simulink model "CH12_1"  (R2021b)
settings: Solver=ode45  StartTime=0.0  StopTime=5  RelTol=1e-3
libraries: dsparch4 x2
settings Model: Creator=NA  LastModifiedBy=IT
settings SolverCC: AlgebraicLoopSolver=TrustRegion
settings DataIOCC: LimitDataPoints=on  SaveFormat=Array  SignalLoggingSaveFormat=ModelDataLogs  ReturnWorkspaceOutputs=off
settings OptimizationCC: BlockReduction=off  BooleanDataType=off  LifeSpan=inf
settings DebuggingCC: SaveWithParameterizedLinksMsg=none  UnderspecifiedInitializationDetection=Classic  MergeDetectMultiDrivingBlocksExec=none  SignalResolutionControl=TryResolveAllWithWarning  FcnCallInpInsideContextMsg=warning  SFUnexpectedBacktrackingDiag=warning  SFNoUnconditionalDefaultTransitionDiag=warning  SFExecutionAtInitializationDiag=none  SFMachineParentedDataDiag=warning  ArithmeticOperatorsInVariantConditions=warning
settings HardwareCC: ProdBitPerPointer=32  ProdBitPerSizeT=32  ProdBitPerPtrDiffT=32  ProdLargestAtomicFloat=None  ProdIntDivRoundTo=Undefined  ProdEndianess=Unspecified  ProdWordSize=32  ProdHWDeviceType=32-bit Generic  TargetUnknown=on
settings ModelReferenceCC: PropagateSignalLabelsOutOfModel=off
settings SFSimCC: SimUseLocalCustomCode=off  CustomCodeUndefinedFunction=UseInterfaceOnly
settings RTWCC: RTWUseLocalCustomCode=off
settings CodeAppCC: StateflowObjectComments=on
settings GRTTargetCC: TargetLangStandard=C89/C90 (ANSI)  CombineOutputUpdateFcns=off  GRTInterface=on
settings ConfigComp: CovMetricSettings=dw  CovSaveCumulativeToWorkspaceVar=on  CovSaveSingleToWorkspaceVar=on  CovExternalEMLEnable=off

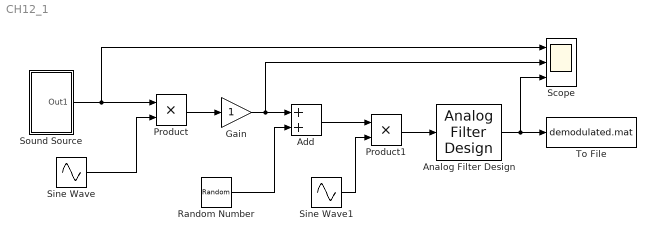
== system CH12_1 ==
  Add : Sum
  Analog Filter Design : dsparch4/Analog Filter Design  method=Butterworth  filttype=Lowpass  N=8  Wlo=2*pi*4e3  Whi=80  Rp=2  Rs=40
  Gain : Gain
  Product : Product
  Product1 : Product
  Random Number : RandomNumber  Variance=1e-6  Seed=41  SampleTime=1/8000  VectorParams1D=off
  Scope : Scope  NumInputPorts=3
  Sine Wave : Sin  Frequency=2*pi*25e3  Phase=pi/2  SampleTime=0
  Sine Wave1 : Sin  Frequency=2*pi*25e3  Phase=pi/2  SampleTime=0
  Sound Source : Subsystem
  To File : ToFile  Filename=demodulated.mat  SampleTime=1/8192
  wires:
  Sound Source/1(Out1) -> Scope/1, Product/1
  Product/1 -> Gain/1
  Gain/1 -> Scope/2, Add/1
  Add/1 -> Product1/1
  Product1/1 -> Analog Filter Design/1
  Analog Filter Design/1 -> Scope/3, To File/1
  Sine Wave/1 -> Product/2
  Random Number/1 -> Add/2
  Sine Wave1/1 -> Product1/2

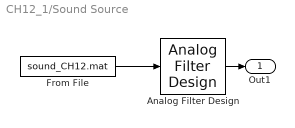
== system CH12_1/Sound Source ==
  Analog Filter Design : dsparch4/Analog Filter Design  method=Butterworth  filttype=Lowpass  N=8  Wlo=2*pi*4e3  Whi=80  Rp=2  Rs=40
  From File : FromFile  FileName=sound_CH12.mat  SampleTime=0
  Out1 : Outport
  wires:
  From File/1 -> Analog Filter Design/1
  Analog Filter Design/1 -> Out1/1
